simulink model "Sistema"  (R2019a)
settings: Solver=VariableStepAuto  StartTime=0.0  StopTime=20  RelTol=1e-3
values from neighbouring files (symbols this model uses):
  kc_IAE = 4    [propeller_levitated_arm.m]
  kc_ISE = 20    [propeller_levitated_arm.m]
  kc_ITAE = 5    [propeller_levitated_arm.m]
  kc_ITSE = 15    [propeller_levitated_arm.m]
  td_IAE = 1.6    [propeller_levitated_arm.m]
  td_ISE = 10    [propeller_levitated_arm.m]
  td_ITAE = 5    [propeller_levitated_arm.m]
  td_ITSE = 6    [propeller_levitated_arm.m]
  ti_IAE = 8    [propeller_levitated_arm.m]
  ti_ISE = 15    [propeller_levitated_arm.m]
  ti_ITAE = 10    [propeller_levitated_arm.m]
  ti_ITSE = 8    [propeller_levitated_arm.m]
settings Model: Creator=julio  LastModifiedBy=julio
settings DataIOCC: SaveOutput=off  SignalLogging=off  DSMLogging=off  SaveTime=off  ReturnWorkspaceOutputs=off  TimeSaveName=time

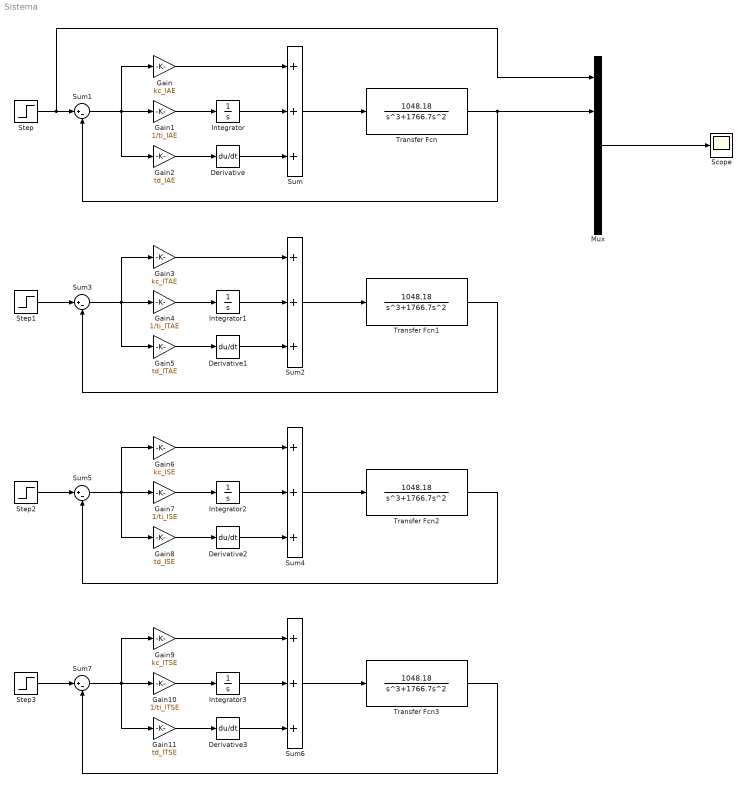
== system Sistema ==
  Derivative{,1..3} (4 alike) : Derivative
  Gain : Gain  Gain=kc_IAE
  Gain1 : Gain  Gain=1/ti_IAE
  Gain10 : Gain  Gain=1/ti_ITSE
  Gain11 : Gain  Gain=td_ITSE
  Gain2 : Gain  Gain=td_IAE
  Gain3 : Gain  Gain=kc_ITAE
  Gain4 : Gain  Gain=1/ti_ITAE
  Gain5 : Gain  Gain=td_ITAE
  Gain6 : Gain  Gain=kc_ISE
  Gain7 : Gain  Gain=1/ti_ISE
  Gain8 : Gain  Gain=td_ISE
  Gain9 : Gain  Gain=kc_ITSE
  Integrator{,1..3} (4 alike) : Integrator
  Mux : Mux  Inputs=5
  Scope : Scope
  Step : Step  SampleTime=1
  Step1 : Step  SampleTime=0
  Step2 : Step  SampleTime=0
  Step3 : Step  SampleTime=0
  Sum{,2,4,6} (4 alike) : Sum  Inputs=+++
  Sum{1,3,5,7} (4 alike) : Sum  Inputs=|+-
  Transfer Fcn{,1..3} (4 alike) : TransferFcn  Numerator=[1048.18]  Denominator=[1 1766.7 0 0]
  wires:
  Gain/1 -> Sum/1
  Gain1/1 -> Integrator/1
  Integrator/1 -> Sum/2
  Gain2/1 -> Derivative/1
  Derivative/1 -> Sum/3
  Sum1/1 -> Gain1/1, Gain2/1, Gain/1
  Sum/1 -> Transfer Fcn/1
  Transfer Fcn/1 -> Sum1/2, Mux/2
  Mux/1 -> Scope/1
  Gain3/1 -> Sum2/1
  Gain4/1 -> Integrator1/1
  Sum2/1 -> Transfer Fcn1/1
  Step1/1 -> Sum3/1
  Integrator1/1 -> Sum2/2
  Sum3/1 -> Gain4/1, Gain5/1, Gain3/1
  Gain5/1 -> Derivative1/1
  Transfer Fcn1/1 -> Sum3/2
  Derivative1/1 -> Sum2/3
  Gain6/1 -> Sum4/1
  Gain7/1 -> Integrator2/1
  Sum4/1 -> Transfer Fcn2/1
  Step2/1 -> Sum5/1
  Integrator2/1 -> Sum4/2
  Sum5/1 -> Gain7/1, Gain8/1, Gain6/1
  Gain8/1 -> Derivative2/1
  Transfer Fcn2/1 -> Sum5/2
  Derivative2/1 -> Sum4/3
  Gain9/1 -> Sum6/1
  Gain10/1 -> Integrator3/1
  Sum6/1 -> Transfer Fcn3/1
  Step3/1 -> Sum7/1
  Integrator3/1 -> Sum6/2
  Sum7/1 -> Gain10/1, Gain11/1, Gain9/1
  Gain11/1 -> Derivative3/1
  Transfer Fcn3/1 -> Sum7/2
  Derivative3/1 -> Sum6/3
  Step/1 -> Mux/1, Sum1/1
